simulink model "Week2Problem1"  (R2020b)
settings: Solver=VariableStepAuto  StartTime=0.0  StopTime=inf  RelTol=1e-3
settings Model: Creator=HP  LastModifiedBy=HP

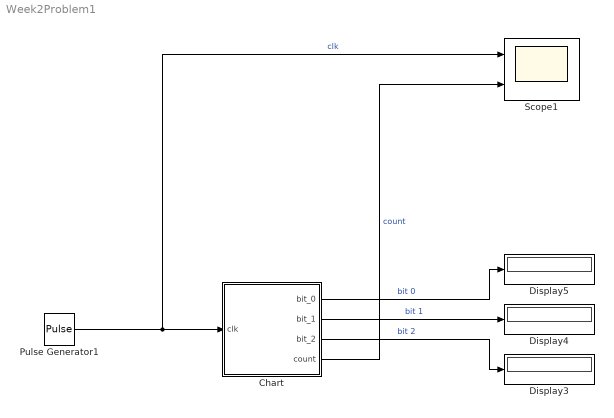
== system Week2Problem1 ==
  Chart : Stateflow chart  TreatAsAtomicUnit=on
  Display3 : Display
  Display4 : Display
  Display5 : Display
  Pulse Generator1 : DiscretePulseGenerator  PulseType=Time based  Period=0.2  PulseWidth=50
  Scope1 : Scope  NumInputPorts=2
  wires:
  Chart/2(bit_1) -> Display4/1  "bit 1"
  Pulse Generator1/1 -> Chart/1(clk), Scope1/1  "clk"
  Chart/1(bit_0) -> Display5/1  "bit 0"
  Chart/4(count) -> Scope1/2  "count"
  Chart/3(bit_2) -> Display3/1  "bit 2"

== stateflow chart Week2Problem1/Chart ==
  state STATE0
    entry:
    bit_0 = 0;
    bit_1 = 0;
    bit_2 = 0;
    exit:
    count = 0;
  state STATE1
    entry:
    bit_0 =1;
    bit_1 = 0;
    bit_2 = 0;
    exit:
    count = 1;
  state STATE5
    entry:
    bit_0=0;
    bit_1=0;
    bit_2=1;
    exit:
    count = 4;
  state STATE2
    entry:
    bit_0 = 0;
    bit_1 = 1;
    bit_2 =0;
    exit:
    count=2;
  state STATE3
    entry:
    bit_0 =1;
    bit_1 =1;
    bit_2 = 0;
    exit:
    count=3;
  (default) -> STATE0
  STATE5 -> STATE0 : [clk==1]
  STATE0 -> STATE1 : [clk==1]
  STATE1 -> STATE2 : [clk==1]
  STATE3 -> STATE5 : [clk==1]
  STATE2 -> STATE3 : [clk==1]
  data: clk input; bit_0 output; bit_1 output; bit_2 output; count output
